simulink model "Human_Fallower_2_R2018b"  (R2018b)
settings: Solver=FixedStepAuto  StartTime=0.0  StopTime=10.0  FixedStep=0.01  RelTol=1e-3
libraries: autolibshared x1, vehdynlibsteering x1
settings Model: Creator=poseidon  LastModifiedBy=ckreienk
settings DataIOCC: ReturnWorkspaceOutputs=on

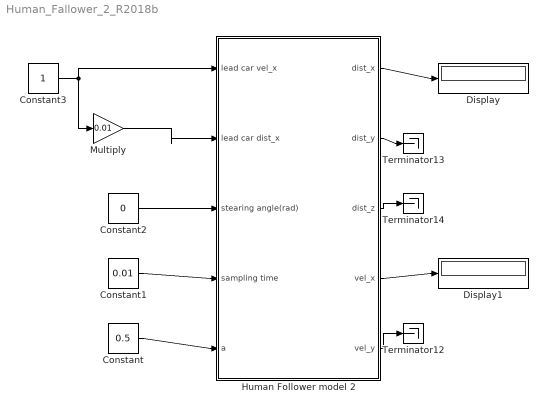
== system Human_Fallower_2_R2018b ==
  Constant : Constant  Value=0.5
  Constant1 : Constant  Value=0.01
  Constant2 : Constant  Value=0
  Constant3 : Constant
  Display : Display
  Display1 : Display
  Human Follower model 2 : Subsystem
  Multiply : Gain  Gain=0.01
  Terminator12 : Terminator
  Terminator13 : Terminator
  Terminator14 : Terminator
  wires:
  Human Follower model 2/2(dist_y) -> Terminator13/1
  Human Follower model 2/3(dist_z) -> Terminator14/1
  Human Follower model 2/5(vel_y) -> Terminator12/1
  Constant/1 -> Human Follower model 2/5(a)
  Constant1/1 -> Human Follower model 2/4(sampling time)
  Constant2/1 -> Human Follower model 2/3(stearing angle(rad))
  Human Follower model 2/1(dist_x) -> Display/1
  Human Follower model 2/4(vel_x) -> Display1/1
  Constant3/1 -> Multiply/1, Human Follower model 2/1(lead car vel_x)
  Multiply/1 -> Human Follower model 2/2(lead car dist_x)

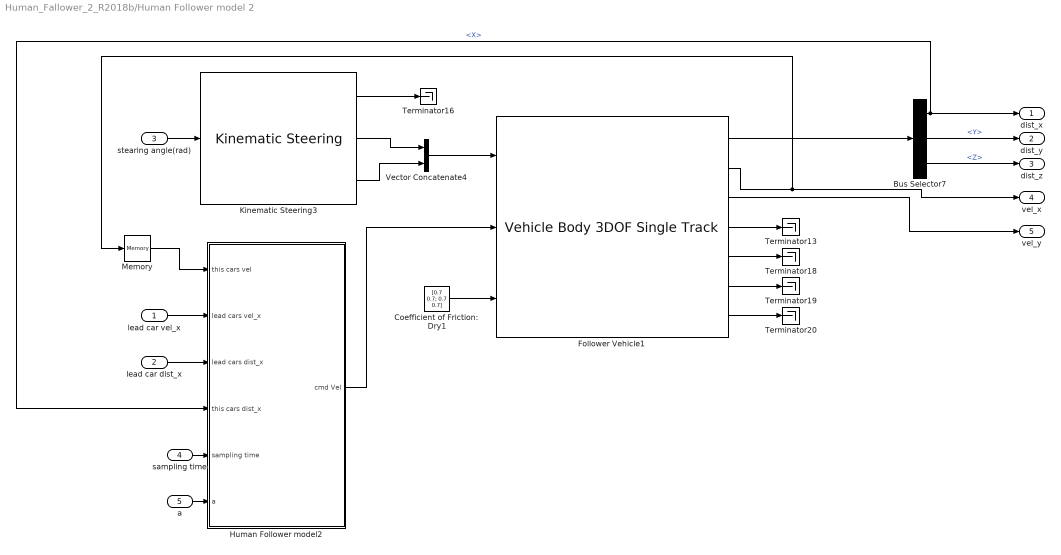
== system Human_Fallower_2_R2018b/Human Follower model 2 ==
  lead car vel_x : Inport
  lead car dist_x : Inport  Port=2
  stearing angle(rad) : Inport  Port=3
  sampling time : Inport  Port=4
  a : Inport  Port=5
  Bus Selector7 : BusSelector  OutputSignals=InertFrm.Cg.Disp.X,InertFrm.Cg.Disp.Y,InertFrm.Cg.Disp.Z
  Coefficient of Friction: Dry1 : Constant  Value=[0.7 0.7; 0.7 0.7]
  Follower Vehicle1 : autolibshared/Vehicle Body 3DOF Single Track  trackMode=Dual  inputMode=External longitudinal velocity  frontSteerMode=on  rearSteerMode=off  windMode=off  muMode=on  extFMode=off  extMMode=off  aMode=2  NF=2  NR=2  m=2000  a=1.4  b=1.6  h=0.35  X_o=0  xdot_o=0  CalphaMode=off  sigmaMode=on  d=0  w=[1.4,1.4]  Cy_f=12e3  Cy_r=11e3  sigma_f=.1  sigma_r=.1  alpha_f_brk=[-.1 .1]  Cy_f_data=[-9e3 9e3]  alpha_r_brk=[-.1 .1]  Cy_r_data=[-9e3 9e3]  Y_o=0  ydot_o=0  Izz=4000  psi_o=0  r_o=0  Af=2  Cd=.3  Cl=.1  Cpm=.1  beta_w=[0:0.01:0.3]  Cs=[0:0.03:0.9]  Cym=[0:0.01:0.3]  Pabs=101325  Tair=273  g=9.81  mu=1  xdot_tol=.01  Fznom=5000  Fxtire_sat=7e4  Fytire_sat=7e4  longOff=0  latOff=0  vertOff=0
      settings: SourceProductName=Powertrain Blockset  SourceProductBaseCode=PW
  Human Follower model2 : Subsystem
  Kinematic Steering3 : vehdynlibsteering/Kinematic Steering  StrgType=Rack and pinion  StrgRatioType=Constant  Loc=Front  NrmlFctr=0.01  TrckWdth=1  WhlBase=1.524  Db=0  StrgRng=1.25*pi  StrgAngBpts="[-6.2832   -5.0265   -3.7699   -2.5133   -1.2566         0    1.2566    2.5133    3.7699    5.0265    6.2832]"  StrgRatioTbl=|  StrgRatio=100  StrgArmLngth=0.1  RckCsLngth=0.5  TieRodLngth=0.248  D=0.2  PnnRadius=0.0057  PnnRadiusTbl="[0.0055    0.0055    0.0056    0.0057    0.0058    0.0057    0.0057    0.0057    0.0056    0.0055    0.0055]"  RodLngth=0.1  ParaArmLngth=0.9  aMode=2
      | [13.5000   13.3750   13.2500   13.1250   13.0000   13.0000   13.0000   13.1250   13.2500   13.3750   13.5000
      | ]
      settings: SourceProductName=Vehicle Dynamics Blockset
  Memory : Memory
  Terminator{13,16,18..20} (5 alike) : Terminator
  Vector Concatenate4 : Concatenate
  dist_x : Outport
  dist_y : Outport  Port=2
  dist_z : Outport  Port=3
  vel_x : Outport  Port=4
  vel_y : Outport  Port=5
  wires:
  Coefficient of Friction: Dry1/1 -> Follower Vehicle1/3
  Follower Vehicle1/2 -> Memory/1, vel_x/1
  Kinematic Steering3/3 -> Vector Concatenate4/2
  stearing angle(rad)/1 -> Kinematic Steering3/1
  Kinematic Steering3/2 -> Vector Concatenate4/1
  Bus Selector7/2 -> dist_y/1  "<Y>"
  Kinematic Steering3/1 -> Terminator16/1
  Follower Vehicle1/1 -> Bus Selector7/1
  Vector Concatenate4/1 -> Follower Vehicle1/1
  Follower Vehicle1/7 -> Terminator20/1
  Follower Vehicle1/3 -> vel_y/1
  Follower Vehicle1/4 -> Terminator13/1
  Bus Selector7/1 -> Human Follower model2/4(this cars dist_x), dist_x/1  "<X>"
  Follower Vehicle1/6 -> Terminator19/1
  Human Follower model2/1(cmd Vel) -> Follower Vehicle1/2
  Follower Vehicle1/5 -> Terminator18/1
  Bus Selector7/3 -> dist_z/1  "<Z>"
  sampling time/1 -> Human Follower model2/5(sampling time)
  a/1 -> Human Follower model2/6(a)
  lead car dist_x/1 -> Human Follower model2/3(lead cars dist_x)
  lead car vel_x/1 -> Human Follower model2/2(lead cars vel_x)
  Memory/1 -> Human Follower model2/1(this cars vel)

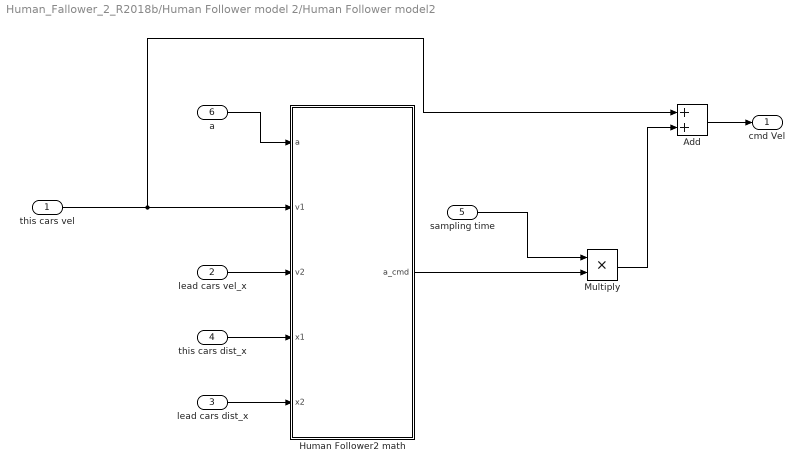
== system Human_Fallower_2_R2018b/Human Follower model 2/Human Follower model2 ==
  this cars vel : Inport
  lead cars vel_x : Inport  Port=2
  lead cars dist_x : Inport  Port=3
  this cars dist_x : Inport  Port=4
  sampling time : Inport  Port=5
  a : Inport  Port=6
  Add : Sum
  Human Follower2 math : Subsystem
  Multiply : Product
  cmd Vel : Outport
  wires:
  sampling time/1 -> Multiply/1
  Multiply/1 -> Add/2
  Human Follower2 math/1(a_cmd) -> Multiply/2
  this cars vel/1 -> Human Follower2 math/2(v1), Add/1
  Add/1 -> cmd Vel/1
  a/1 -> Human Follower2 math/1(a)
  lead cars dist_x/1 -> Human Follower2 math/5(x2)
  lead cars vel_x/1 -> Human Follower2 math/3(v2)
  this cars dist_x/1 -> Human Follower2 math/4(x1)

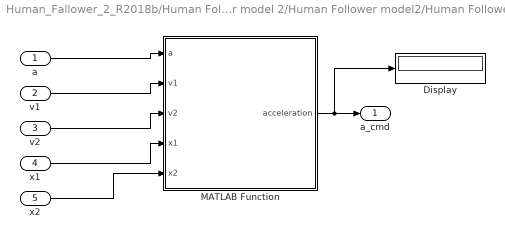
== system Human_Fallower_2_R2018b/Human Follower model 2/Human Follower model2/Human Follower2 math ==
  a : Inport
  v1 : Inport  Port=2
  v2 : Inport  Port=3
  x1 : Inport  Port=4
  x2 : Inport  Port=5
  Display : Display
  MATLAB Function : MATLAB Function  TreatAsAtomicUnit=on
  a_cmd : Outport
  wires:
  v1/1 -> MATLAB Function/2(v1)
  a/1 -> MATLAB Function/1(a)
  v2/1 -> MATLAB Function/3(v2)
  MATLAB Function/1(acceleration) -> Display/1, a_cmd/1
  x1/1 -> MATLAB Function/4(x1)
  x2/1 -> MATLAB Function/5(x2)

== matlab function Human_Fallower_2_R2018b/Human Follower model 2/Human Follower model2/Human Follower2 math/MATLAB Function ==
  data: a input; v1 input; v2 input; x1 input; acceleration output; x2 input
function acceleration = fcn(a, v1, v2, x1, x2)


if x2 == 0
    x2 = 0.1;
end

acceleration = a*(v2 - v1) / (x2 - x1);
